simulink model "linearized"  (R2024b)
settings: Solver=ode4  StartTime=0.0  StopTime=StopTime  FixedStep=StepSize  RelTol=1e-3
values from neighbouring files (symbols this model uses):
  A = zeros(9,9)    [state_space.m]
  B = zeros(9,3)    [state_space.m]
  C = eye(9)    [state_space.m]
  D = zeros(9,3)    [state_space.m]
  initial_conditions = [      V0,      gamma0,      R0,      p0,      q0,      r0,      alpha0,      beta0,      sigma0  ]    [state_space.m]
  Mars_radius = 6371e3    (= 6371000)    [state_space.m]
undefined symbols (not defined in the file or in its folder): K_lqr
settings Model: Creator=rafae  LastModifiedBy=rafae
settings DataIOCC: ReturnWorkspaceOutputs=off

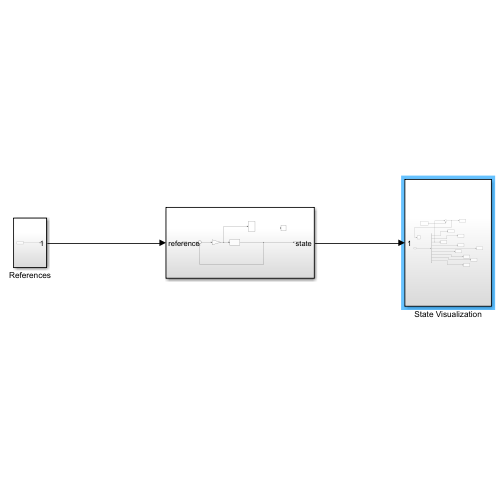
[thumbnail: Simulink's stored preview of the top-level diagram]
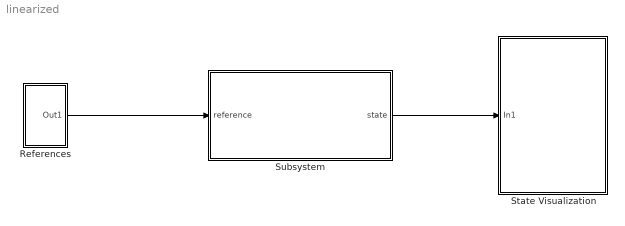
== system linearized ==
  References : Subsystem
  State Visualization : Subsystem
  Subsystem : Subsystem
  wires:
  Subsystem/1(state) -> State Visualization/1(In1)
  References/1(Out1) -> Subsystem/1(reference)

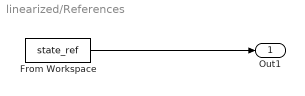
== system linearized/References ==
  From Workspace : FromWorkspace  VariableName=state_ref
  Out1 : Outport
  wires:
  From Workspace/1 -> Out1/1

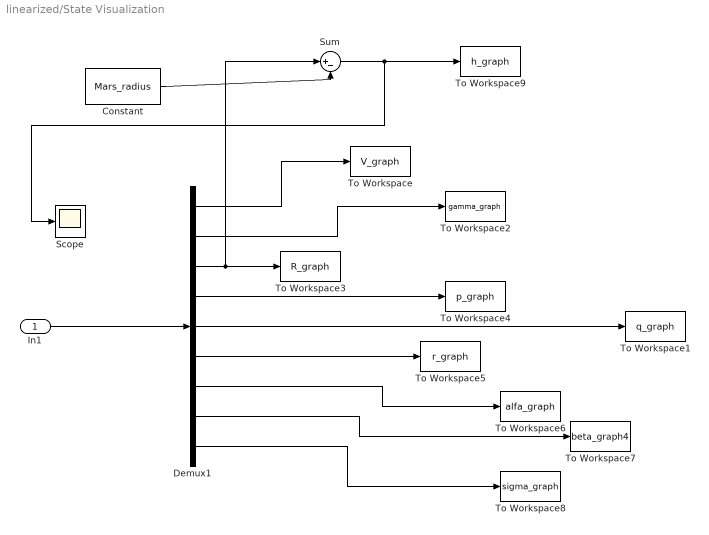
== system linearized/State Visualization ==
  In1 : Inport
  Constant : Constant  Value=Mars_radius
  Demux1 : Demux  Outputs=9
  Scope : Scope
  Sum : Sum  Inputs=|+-
  To Workspace : ToWorkspace  VariableName=V_graph  SaveFormat=Structure With Time  SampleTime=-1
  To Workspace1 : ToWorkspace  VariableName=q_graph  SaveFormat=Structure With Time  SampleTime=-1
  To Workspace2 : ToWorkspace  VariableName=gamma_graph  SaveFormat=Structure With Time  SampleTime=-1
  To Workspace3 : ToWorkspace  VariableName=R_graph  SaveFormat=Structure With Time  SampleTime=-1
  To Workspace4 : ToWorkspace  VariableName=p_graph  SaveFormat=Structure With Time  SampleTime=-1
  To Workspace5 : ToWorkspace  VariableName=r_graph  SaveFormat=Structure With Time  SampleTime=-1
  To Workspace6 : ToWorkspace  VariableName=alfa_graph  SaveFormat=Structure With Time  SampleTime=-1
  To Workspace7 : ToWorkspace  VariableName=beta_graph4  SaveFormat=Structure With Time  SampleTime=-1
  To Workspace8 : ToWorkspace  VariableName=sigma_graph  SaveFormat=Structure With Time  SampleTime=-1
  To Workspace9 : ToWorkspace  VariableName=h_graph  SaveFormat=Structure With Time  SampleTime=-1
  wires:
  Demux1/5 -> To Workspace1/1
  Demux1/2 -> To Workspace2/1
  Demux1/1 -> To Workspace/1
  Demux1/4 -> To Workspace4/1
  Demux1/8 -> To Workspace7/1
  Demux1/3 -> Sum/1, To Workspace3/1
  Demux1/9 -> To Workspace8/1
  In1/1 -> Demux1/1
  Demux1/7 -> To Workspace6/1
  Demux1/6 -> To Workspace5/1
  Constant/1 -> Sum/2
  Sum/1 -> Scope/1, To Workspace9/1

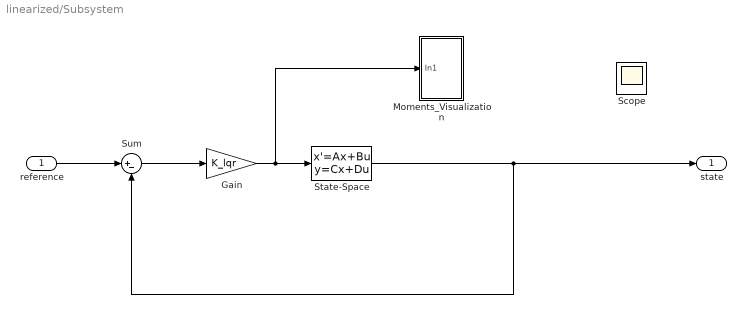
== system linearized/Subsystem ==
  reference : Inport
  Gain : Gain  Gain=K_lqr
  Moments_Visualization : Subsystem
  Scope : Scope
  State-Space : StateSpace  A=A  B=B  C=C  D=D  InitialCondition=initial_conditions
  Sum : Sum  Inputs=|+-
  state : Outport
  wires:
  State-Space/1 -> Sum/2, state/1
  reference/1 -> Sum/1
  Sum/1 -> Gain/1
  Gain/1 -> Moments_Visualization/1(In1), State-Space/1

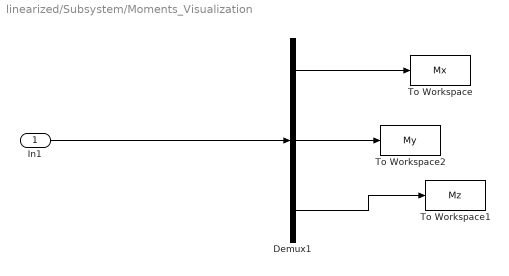
== system linearized/Subsystem/Moments_Visualization ==
  In1 : Inport
  Demux1 : Demux  Outputs=3
  To Workspace : ToWorkspace  VariableName=Mx  SaveFormat=Structure With Time  SampleTime=-1
  To Workspace1 : ToWorkspace  VariableName=Mz  SaveFormat=Structure With Time  SampleTime=-1
  To Workspace2 : ToWorkspace  VariableName=My  SaveFormat=Structure With Time  SampleTime=-1
  wires:
  Demux1/2 -> To Workspace2/1
  Demux1/1 -> To Workspace/1
  In1/1 -> Demux1/1
  Demux1/3 -> To Workspace1/1
